simulink model "bms2"  (R2017b)
settings: Solver=VariableStepAuto  StartTime=0.0  StopTime=600  MaxStep=1e-4  RelTol=1e-3
undefined symbols (not defined in the file): Hydride, Metal, Nickel
libraries: powerlib x11, electricdrivelib x3
settings Model: Creator=DELL  LastModifiedBy=DELL

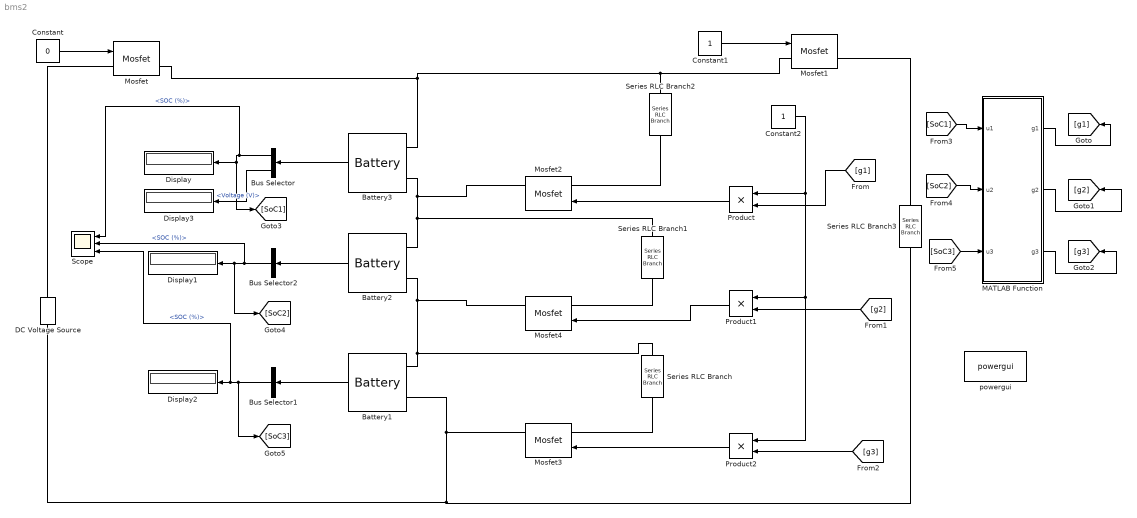
== system bms2 ==
  Battery1 : electricdrivelib/Extra Sources/Battery  BatType=Nickel-Metal-Hydride  ShowTempParam=on  ThermalPreset="3.6V  2050mAh   (LiCoO2)"  ShowAgeParam=off  NomV=7.2  NomQ=6.5  SOC=68  Batt_Tr=1  PresetModel=on  MaxQ=7  MinV=5.4  FullV=8.4814  Dis_rate=1.3  R=0.011077  Normal_OP=6.25  expZone="[7.8102         1.3]"  current=[6.5 13 32.5]  Units=Time  Tci=20  NomT=25  T2=0  MaxQ2=1.78  FullV2=4  Normal_OP2=3.11  expZone2="[3.8         0.2]"  Rca=0.06  ti=1000  Dp=0  Neq0=0  Tsim=1e6  Ta1=25  Qeol=5.4*0.9  Reol=0.013333*1.2  Char_age=[2.3478, 3]  Dis_age=[2.3478, 10]  N1=1500  N2=10500  N3=1000  N4=1400  Ta2=45  N5=950
  Battery2 : electricdrivelib/Extra Sources/Battery  BatType=Nickel-Metal-Hydride  ShowTempParam=on  ThermalPreset="3.6V  2050mAh   (LiCoO2)"  ShowAgeParam=off  NomV=7.2  NomQ=6.5  SOC=65  Batt_Tr=1  PresetModel=on  MaxQ=7  MinV=5.4  FullV=8.4814  Dis_rate=1.3  R=0.011077  Normal_OP=6.25  expZone="[7.8102         1.3]"  current=[6.5 13 32.5]  Units=Time  Tci=20  NomT=25  T2=0  MaxQ2=1.78  FullV2=4  Normal_OP2=3.11  expZone2="[3.8         0.2]"  Rca=0.06  ti=1000  Dp=0  Neq0=0  Tsim=1e6  Ta1=25  Qeol=5.4*0.9  Reol=0.013333*1.2  Char_age=[2.3478, 3]  Dis_age=[2.3478, 10]  N1=1500  N2=10500  N3=1000  N4=1400  Ta2=45  N5=950
  Battery3 : electricdrivelib/Extra Sources/Battery  BatType=Nickel-Metal-Hydride  ShowTempParam=on  ThermalPreset="3.6V  2050mAh   (LiCoO2)"  ShowAgeParam=off  NomV=7.2  NomQ=6.5  SOC=60  Batt_Tr=1  PresetModel=on  MaxQ=7  MinV=5.4  FullV=8.4814  Dis_rate=1.3  R=0.011077  Normal_OP=6.25  expZone="[7.8102         1.3]"  current=[6.5 13 32.5]  Units=Time  Tci=20  NomT=25  T2=0  MaxQ2=1.78  FullV2=4  Normal_OP2=3.11  expZone2="[3.8         0.2]"  Rca=0.06  ti=1000  Dp=0  Neq0=0  Tsim=1e6  Ta1=25  Qeol=5.4*0.9  Reol=0.013333*1.2  Char_age=[2.3478, 3]  Dis_age=[2.3478, 10]  N1=1500  N2=10500  N3=1000  N4=1400  Ta2=45  N5=950
  Bus Selector : BusSelector  OutputSignals=SOC (%),Voltage (V)
  Bus Selector1 : BusSelector  OutputSignals=SOC (%)
  Bus Selector2 : BusSelector  OutputSignals=SOC (%)
  Constant : Constant  Value=0
  Constant1 : Constant
  Constant2 : Constant
  DC Voltage Source : powerlib/Electrical Sources/DC Voltage Source  Amplitude=27  Measurements=Voltage
  Display{,1..3} (4 alike) : Display
  MATLAB Function : MATLAB Function  TreatAsAtomicUnit=on
  Mosfet{,1..4} (5 alike) : powerlib/Power Electronics/Mosfet  Ron=0.1  Lon=0  Rd=0.01  Vfd=0  IC=0  Rs=1e5  Cs=inf  Measurements=on
  Product : Product
  Product1 : Product
  Product2 : Product
  Scope : Scope  NumInputPorts=3
  Series RLC Branch{,1..3} (4 alike) : powerlib/Elements/Series RLC Branch  LConnTagsString=__new0  RConnTagsString=__new0  BranchType=R  Resistance=1  Inductance=1e-3  SetiL0=off  InitialCurrent=0  Capacitance=1e-6  Setx0=off  InitialVoltage=0  Measurements=None
  powergui : powerlib/powergui  Priority=1  SimulationMode=Continuous  SampleTime=50e-6  frequency=60  Iterations=50  frequencyindice=0  Pbase=100e6  ErrMax=1e-4  UnitsV=kV  UnitsW=MW  buscounter=0  FunctionMessages=off  echomessages=off  EnableUseOfTLC=off  CurrentSourceSwitches=off  DisableSnubberDevices=off  DisableRonSwitches=off  DisableVfSwitches=off  DisplayEquations=off  SolverType=Tustin/Backward Euler (TBE)  Interpol=off  ExternalGateDelay=off  methode=off  Ts=100  x0status=blocks  SPID=on  SwTol=0  HookPort=off  RestoreLinks=warning  ResistiveCurrentMeasurement=off  Frange=[0:2:500]  Ylog=off  Xlog=on  ShowGrid=off  save=off  variable=ZData  structure=0  ZoomFFT=off  StartTime=0.0  cycles=1  DisplayStyle=1  fundamental=60  FreqAxis=off  MaxFrequency=1000  frequencyindicesteady=1  RmsSteady=1  display=off
  wires:
  Battery3/1 -> Bus Selector/1
  Battery2/1 -> Bus Selector2/1
  Battery1/1 -> Bus Selector1/1
  Bus Selector/1 -> Scope/1, [SoC1], Display/1  "<SOC (%)>"
  Bus Selector2/1 -> Scope/2, [SoC2], Display1/1  "<SOC (%)>"
  Bus Selector1/1 -> [SoC3], Scope/3, Display2/1  "<SOC (%)>"
  Constant2/1 -> Product/1, Product1/1, Product2/1
  [g1] -> Product/2
  [g2] -> Product1/2
  [g3] -> Product2/2
  MATLAB Function/1(g1) -> [g1]
  MATLAB Function/2(g2) -> [g2]
  MATLAB Function/3(g3) -> [g3]
  [SoC1] -> MATLAB Function/1(u1)
  [SoC2] -> MATLAB Function/2(u2)
  [SoC3] -> MATLAB Function/3(u3)
  Constant/1 -> Mosfet/1
  Constant1/1 -> Mosfet1/1
  Product/1 -> Mosfet2/1
  Product1/1 -> Mosfet4/1
  Product2/1 -> Mosfet3/1
  Bus Selector/2 -> Display3/1  "<Voltage (V)>"
  connections:
  Battery2/LConn1 -- Battery3/LConn2 -- Mosfet2/RConn1 -- Series RLC Branch1/LConn1
  Battery2/LConn2 -- Mosfet4/RConn1 -- Series RLC Branch/LConn1 -- Battery1/LConn1
  Battery1/LConn2 -- Mosfet3/RConn1 -- DC Voltage Source/LConn1 -- Series RLC Branch3/RConn1
  Series RLC Branch2/LConn1 -- Mosfet1/LConn1 -- Battery3/LConn1 -- Mosfet/RConn1
  DC Voltage Source/RConn1 -- Mosfet/LConn1
  Mosfet1/RConn1 -- Series RLC Branch3/LConn1
  Mosfet2/LConn1 -- Series RLC Branch2/RConn1
  Mosfet4/LConn1 -- Series RLC Branch1/RConn1
  Mosfet3/LConn1 -- Series RLC Branch/RConn1

== matlab function bms2/MATLAB Function ==
  data: u1 input; g1 output; u2 input; u3 input; g2 output; g3 output
function [g1,g2,g3] = fcn(u1,u2,u3)

u1 = u1*1000;
u2 = u2*1000;
u3 = u3*1000;

u1 = int32(u1);
u2 = int32(u2);
u3 = int32(u3);

if u1>u2 || u1>u3
     g1 = 1
else
     g1 = 0
end

if u2>u1 || u2>u3
     g2 = 1
else
     g2 = 0
end

if u3>u1 || u3>u2
     g3 = 1
else
     g3 = 0
end

end
